simulink model "univshiftreg"  (R2020a)
settings: Solver=VariableStepAuto  StartTime=0.0  StopTime=10.0  RelTol=1e-3
libraries: simulink_extras x4, dspsrcs4 x1
settings Model: Creator=kishan  LastModifiedBy=kishan

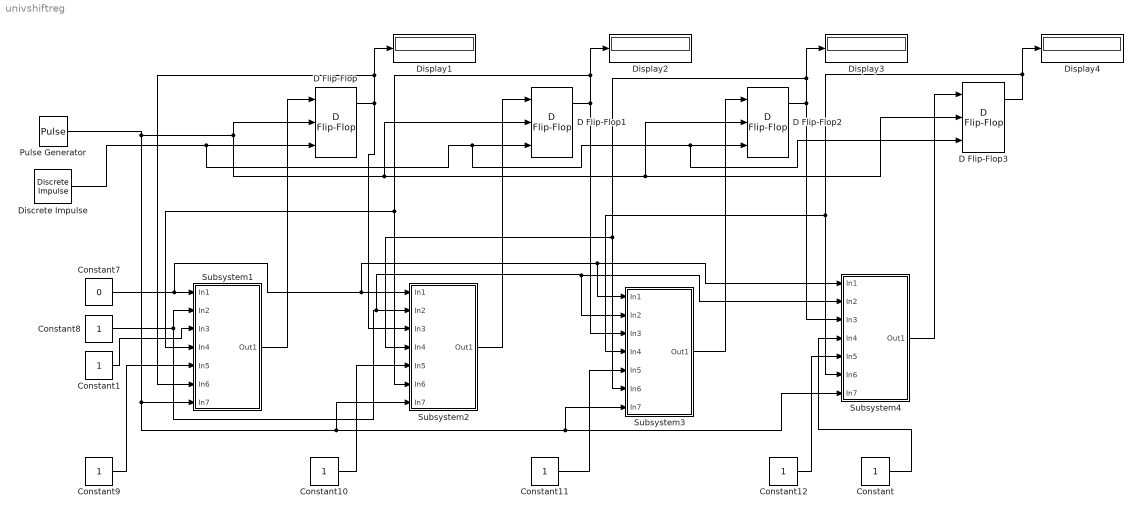
== system univshiftreg ==
  Constant{,1,8..12} (7 alike) : Constant
  Constant7 : Constant  Value=0
  D Flip-Flop{,1..3} (4 alike) : simulink_extras/Flip Flops/D Flip-Flop
  Discrete Impulse : dspsrcs4/Discrete  Impulse  Delay=0  SampleTime=1  FrameSample=1  OutputFrames=off  dataType=double  isSigned=on  wordLen=16  udDataType=sfix(16)  fracBitsMode=Best precision  numFracBits=15  OutDataTypeStr=double  LastOutDataTypeStr=double
  Display{1..4} (4 alike) : Display
  Pulse Generator : DiscretePulseGenerator  PulseType=Time based  Period=10  PulseWidth=5
  Subsystem1 : Subsystem
  Subsystem2 : Subsystem
  Subsystem3 : Subsystem
  Subsystem4 : Subsystem
  wires:
  Subsystem3/1(Out1) -> D Flip-Flop2/1
  Subsystem4/1(Out1) -> D Flip-Flop3/1
  Subsystem2/1(Out1) -> D Flip-Flop1/1
  Subsystem1/1(Out1) -> D Flip-Flop/1
  Pulse Generator/1 -> Subsystem4/7(In7), Subsystem3/7(In7), Subsystem2/7(In7), Subsystem1/7(In7), D Flip-Flop/2, D Flip-Flop1/2, D Flip-Flop3/2, D Flip-Flop2/2
  D Flip-Flop3/1 -> Display4/1, Subsystem3/4(In4), Subsystem4/6(In6)
  D Flip-Flop2/1 -> Subsystem4/3(In3), Display3/1, Subsystem2/4(In4), Subsystem3/6(In6)
  D Flip-Flop1/1 -> Subsystem3/3(In3), Display2/1, Subsystem1/4(In4), Subsystem2/6(In6)
  D Flip-Flop/1 -> Subsystem2/3(In3), Display1/1, Subsystem1/6(In6)
  Constant7/1 -> Subsystem3/1(In1), Subsystem4/1(In1), Subsystem2/1(In1), Subsystem1/1(In1)
  Constant8/1 -> Subsystem1/2(In2), Subsystem4/2(In2), Subsystem3/2(In2), Subsystem2/2(In2)
  Constant12/1 -> Subsystem4/5(In5)
  Constant11/1 -> Subsystem3/5(In5)
  Constant10/1 -> Subsystem2/5(In5)
  Constant9/1 -> Subsystem1/5(In5)
  Constant/1 -> Subsystem4/4(In4)
  Constant1/1 -> Subsystem1/3(In3)
  Discrete Impulse/1 -> D Flip-Flop3/3, D Flip-Flop2/3, D Flip-Flop1/3, D Flip-Flop/3

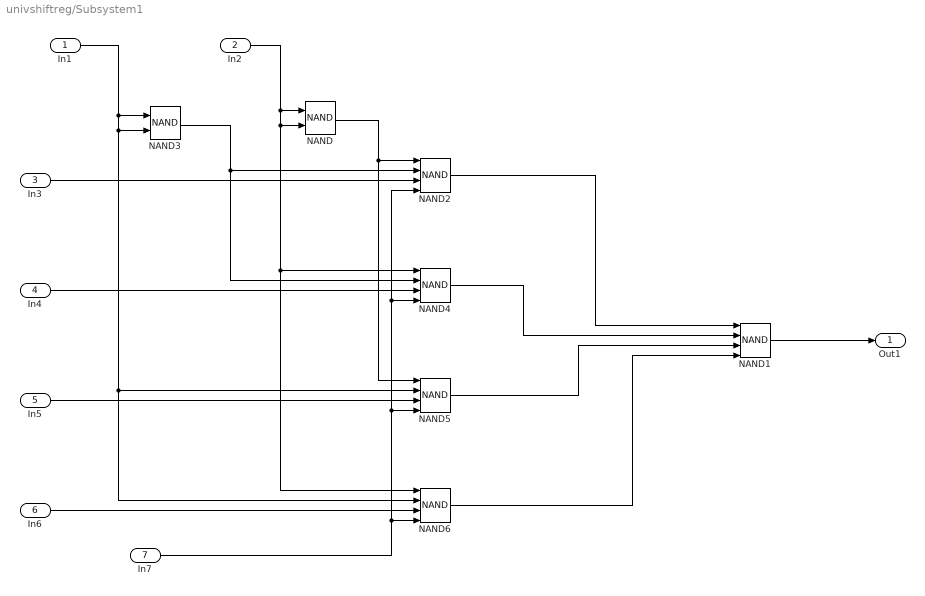
== system univshiftreg/Subsystem1 ==
  In1 : Inport
  In2 : Inport  Port=2
  In3 : Inport  Port=3
  In4 : Inport  Port=4
  In5 : Inport  Port=5
  In6 : Inport  Port=6
  In7 : Inport  Port=7
  NAND : Logic  Operator=NAND  AllPortsSameDT=off  OutDataTypeStr=boolean
  NAND{1..2,4..6} (5 alike) : Logic  Operator=NAND  Inputs=4  AllPortsSameDT=off  OutDataTypeStr=boolean
  NAND3 : Logic  Operator=NAND  AllPortsSameDT=off  OutDataTypeStr=boolean
  Out1 : Outport
  wires:
  NAND6/1 -> NAND1/4
  In5/1 -> NAND5/3
  NAND3/1 -> NAND4/2, NAND2/2
  In1/1 -> NAND6/2, NAND5/2, NAND3/2, NAND3/1
  In2/1 -> NAND6/1, NAND4/1, NAND/2, NAND/1
  In4/1 -> NAND4/3
  In3/1 -> NAND2/3
  NAND/1 -> NAND5/1, NAND2/1
  NAND1/1 -> Out1/1
  In6/1 -> NAND6/3
  NAND5/1 -> NAND1/3
  NAND4/1 -> NAND1/2
  In7/1 -> NAND2/4, NAND4/4, NAND5/4, NAND6/4
  NAND2/1 -> NAND1/1

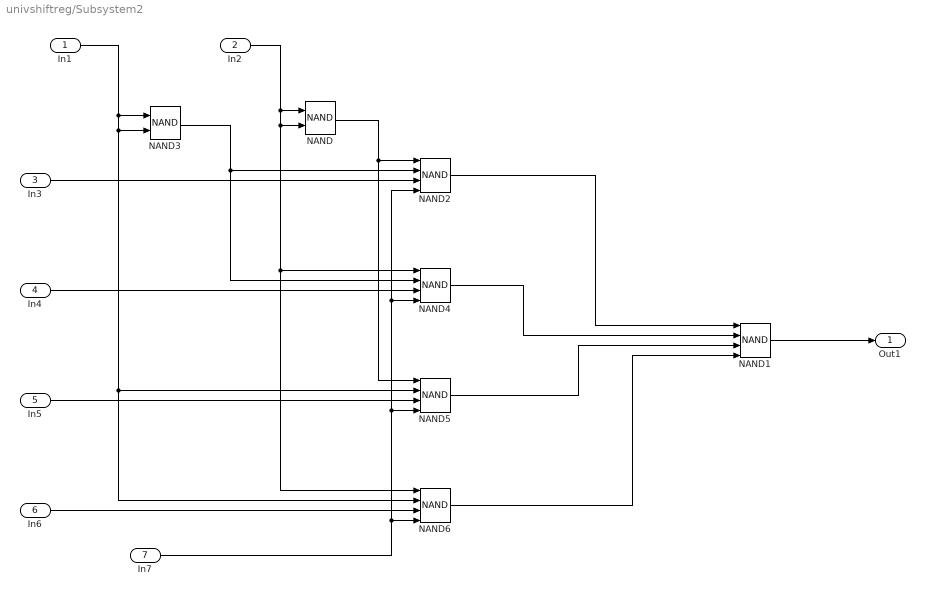
== system univshiftreg/Subsystem2 ==
  In1 : Inport
  In2 : Inport  Port=2
  In3 : Inport  Port=3
  In4 : Inport  Port=4
  In5 : Inport  Port=5
  In6 : Inport  Port=6
  In7 : Inport  Port=7
  NAND : Logic  Operator=NAND  AllPortsSameDT=off  OutDataTypeStr=boolean
  NAND{1..2,4..6} (5 alike) : Logic  Operator=NAND  Inputs=4  AllPortsSameDT=off  OutDataTypeStr=boolean
  NAND3 : Logic  Operator=NAND  AllPortsSameDT=off  OutDataTypeStr=boolean
  Out1 : Outport
  wires:
  NAND6/1 -> NAND1/4
  In5/1 -> NAND5/3
  NAND3/1 -> NAND4/2, NAND2/2
  In1/1 -> NAND6/2, NAND5/2, NAND3/2, NAND3/1
  In2/1 -> NAND6/1, NAND4/1, NAND/2, NAND/1
  In4/1 -> NAND4/3
  In3/1 -> NAND2/3
  NAND/1 -> NAND5/1, NAND2/1
  NAND1/1 -> Out1/1
  In6/1 -> NAND6/3
  NAND5/1 -> NAND1/3
  NAND4/1 -> NAND1/2
  In7/1 -> NAND2/4, NAND4/4, NAND5/4, NAND6/4
  NAND2/1 -> NAND1/1

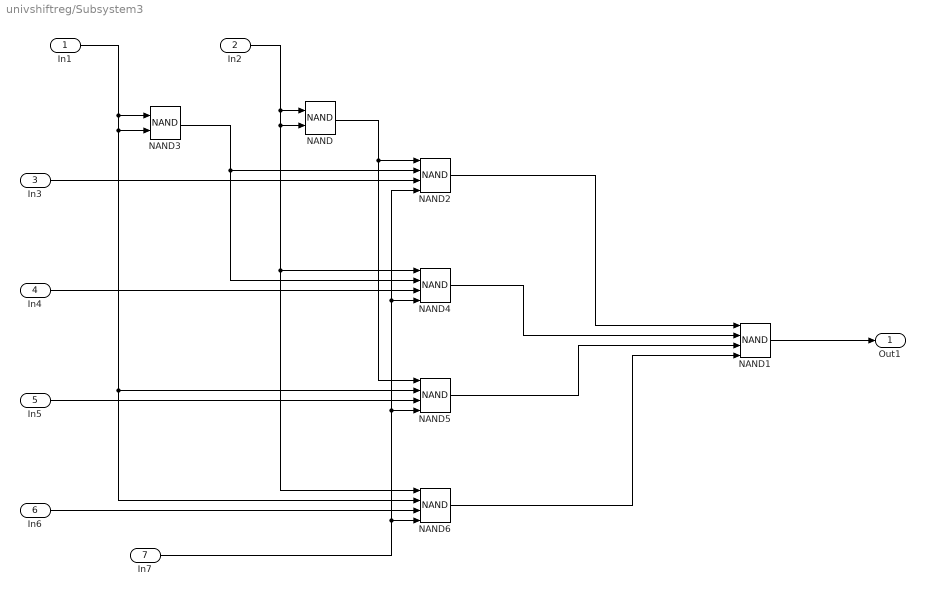
== system univshiftreg/Subsystem3 ==
  In1 : Inport
  In2 : Inport  Port=2
  In3 : Inport  Port=3
  In4 : Inport  Port=4
  In5 : Inport  Port=5
  In6 : Inport  Port=6
  In7 : Inport  Port=7
  NAND : Logic  Operator=NAND  AllPortsSameDT=off  OutDataTypeStr=boolean
  NAND{1..2,4..6} (5 alike) : Logic  Operator=NAND  Inputs=4  AllPortsSameDT=off  OutDataTypeStr=boolean
  NAND3 : Logic  Operator=NAND  AllPortsSameDT=off  OutDataTypeStr=boolean
  Out1 : Outport
  wires:
  NAND6/1 -> NAND1/4
  In5/1 -> NAND5/3
  NAND3/1 -> NAND4/2, NAND2/2
  In1/1 -> NAND6/2, NAND5/2, NAND3/2, NAND3/1
  In2/1 -> NAND6/1, NAND4/1, NAND/2, NAND/1
  In4/1 -> NAND4/3
  In3/1 -> NAND2/3
  NAND/1 -> NAND5/1, NAND2/1
  NAND1/1 -> Out1/1
  In6/1 -> NAND6/3
  NAND5/1 -> NAND1/3
  NAND4/1 -> NAND1/2
  In7/1 -> NAND2/4, NAND4/4, NAND5/4, NAND6/4
  NAND2/1 -> NAND1/1

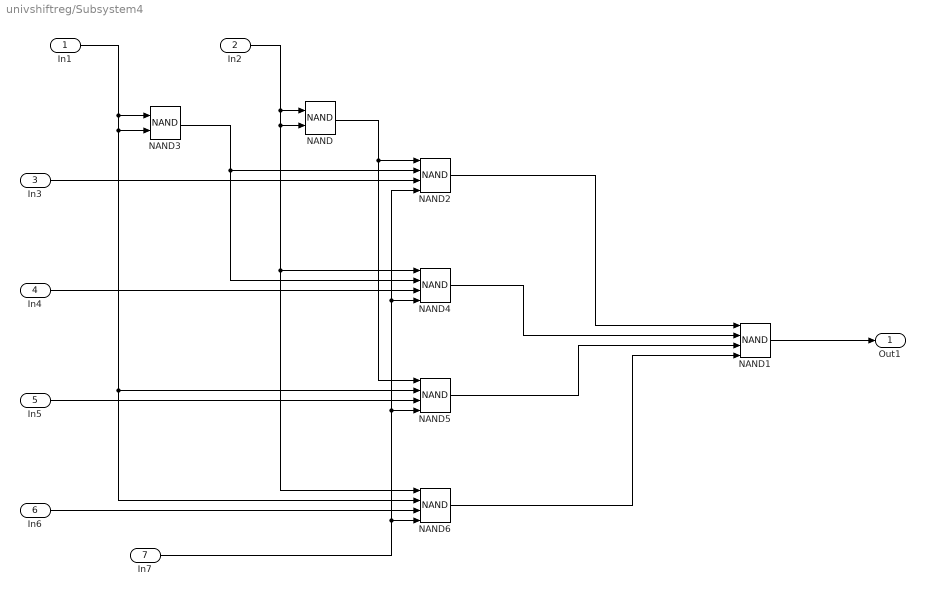
== system univshiftreg/Subsystem4 ==
  In1 : Inport
  In2 : Inport  Port=2
  In3 : Inport  Port=3
  In4 : Inport  Port=4
  In5 : Inport  Port=5
  In6 : Inport  Port=6
  In7 : Inport  Port=7
  NAND : Logic  Operator=NAND  AllPortsSameDT=off  OutDataTypeStr=boolean
  NAND{1..2,4..6} (5 alike) : Logic  Operator=NAND  Inputs=4  AllPortsSameDT=off  OutDataTypeStr=boolean
  NAND3 : Logic  Operator=NAND  AllPortsSameDT=off  OutDataTypeStr=boolean
  Out1 : Outport
  wires:
  NAND6/1 -> NAND1/4
  In5/1 -> NAND5/3
  NAND3/1 -> NAND4/2, NAND2/2
  In1/1 -> NAND6/2, NAND5/2, NAND3/2, NAND3/1
  In2/1 -> NAND6/1, NAND4/1, NAND/2, NAND/1
  In4/1 -> NAND4/3
  In3/1 -> NAND2/3
  NAND/1 -> NAND5/1, NAND2/1
  NAND1/1 -> Out1/1
  In6/1 -> NAND6/3
  NAND5/1 -> NAND1/3
  NAND4/1 -> NAND1/2
  In7/1 -> NAND2/4, NAND4/4, NAND5/4, NAND6/4
  NAND2/1 -> NAND1/1
